simulink model "controltrayectorias"  (R2024b)
settings: Solver=VariableStepAuto  StartTime=0.0  StopTime=10.0  RelTol=1e-3
undefined symbols (not defined in the file or in its folder): matriz3x3
settings Model: Creator=gabyc  LastModifiedBy=gabyc

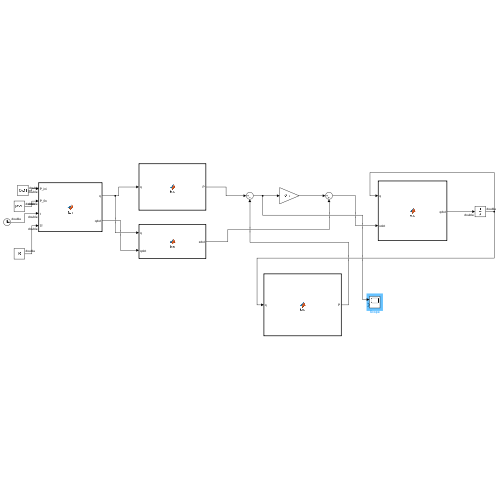
[thumbnail: Simulink's stored preview of the top-level diagram]
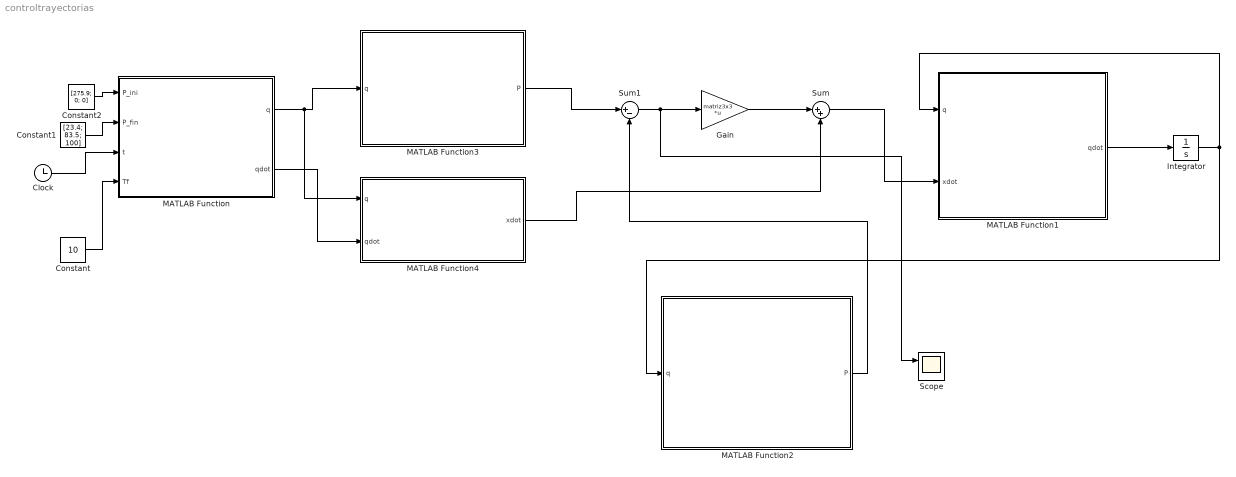
== system controltrayectorias ==
  Clock : Clock
  Constant : Constant  Value=10
  Constant1 : Constant  Value=[23.4; 83.5; 100]
  Constant2 : Constant  Value=[275.9; 0; 0]
  Gain : Gain  Gain=matriz3x3  Multiplication=Matrix(K*u)
  Integrator : Integrator
  MATLAB Function : MATLAB Function  TreatAsAtomicUnit=on
  MATLAB Function1 : MATLAB Function  TreatAsAtomicUnit=on
  MATLAB Function2 : MATLAB Function  TreatAsAtomicUnit=on
  MATLAB Function3 : MATLAB Function  TreatAsAtomicUnit=on
  MATLAB Function4 : MATLAB Function  TreatAsAtomicUnit=on
  Scope : Scope  NumInputPorts=2
  Sum : Sum  Inputs=|++
  Sum1 : Sum  Inputs=|+-
  wires:
  Sum1/1 -> Scope/1, Gain/1
  Gain/1 -> Sum/1
  MATLAB Function1/1(qdot) -> Integrator/1
  Sum/1 -> MATLAB Function1/2(xdot)
  Integrator/1 -> MATLAB Function2/1(q), MATLAB Function1/1(q)
  MATLAB Function2/1(P) -> Sum1/2
  Constant/1 -> MATLAB Function/4(Tf)
  Constant1/1 -> MATLAB Function/2(P_fin)
  Constant2/1 -> MATLAB Function/1(P_ini)
  Clock/1 -> MATLAB Function/3(t)
  MATLAB Function/1(q) -> MATLAB Function4/1(q), MATLAB Function3/1(q)
  MATLAB Function3/1(P) -> Sum1/1
  MATLAB Function/2(qdot) -> MATLAB Function4/2(qdot)
  MATLAB Function4/1(xdot) -> Sum/2

== matlab function controltrayectorias/MATLAB Function1 ==
  data: q input double size=[3 1]; qdot output double size=[3 1]; xdot input double size=[3 1]

function qdot = fcn(q, xdot)
% ============================================================
% Bloque MATLAB Function para Simulink
% Calcula las velocidades articulares qdot = Jinv(q) * xdot
%
% Entradas:
%   q     = [3x1] vector de posiciones articulares
%   xdot  = [3x1] vector de velocidades cartesianas
%
% Salida:
%   qdot  = [3x1] vector de velocidades articulares
% ============================================================


% Llamada a la función del Jacobiano inverso
Jinv = JacInv_PRR(q)

% Multiplicación matricial
qdot = Jinv * xdot;

end

== matlab function controltrayectorias/MATLAB Function ==
  data: P_ini input size=[3 1]; q output size=[3 1]; P_fin input size=[3 1]; t input size=[1 1]; Tf input size=[1 1]; qdot output size=[3 1]
function [q, qdot] = fcn(P_ini, P_fin, t, Tf)
[q, qdot] = trayectoriaCubica_PRR(P_ini, P_fin, t, Tf);
end

== matlab function controltrayectorias/MATLAB Function2 ==
  data: P output double size=[3 1]; q input double size=[3 1]
function P = fcn(q)
%#codegen


P = cinematica_directa(q);

end

== matlab function controltrayectorias/MATLAB Function3 ==
  data: P output double size=[3 1]; q input double size=[3 1]
function P = fcn(q)
%#codegen
P = cinematica_directa(q);
end

== matlab function controltrayectorias/MATLAB Function4 ==
  data: q input; xdot output size=[3 1]; qdot input size=[3 1]
function xdot = fcn(q,qdot)
%#codegen
xdot = velocidadPRR(q, qdot)
end
